simulink model "bus_io"  (Simulink 10.1)
settings: Solver=FixedStepDiscrete  StartTime=0.0  StopTime=10.0  RelTol=1e-3  EnableMultiTasking=on
settings Model: Creator=Demo  LastModifiedBy=MaximeBe
settings DataIOCC: LimitDataPoints=on  SaveFormat=Dataset
settings OptimizationCC: ZeroExternalMemoryAtStartup=off  ZeroInternalMemoryAtStartup=off  LifeSpan=auto
settings DebuggingCC: UnderspecifiedInitializationDetection=Simplified  MergeDetectMultiDrivingBlocksExec=error  AllowSymbolicDim=off  SFExecutionAtInitializationDiag=warning
settings HardwareCC: ProdBitPerPointer=64  ProdBitPerSizeT=64  ProdBitPerPtrDiffT=64  ProdLargestAtomicFloat=Float  ProdIntDivRoundTo=Zero  ProdEndianess=LittleEndian  ProdWordSize=64  ProdHWDeviceType=Intel->x86-64 (Windows64)
settings RTWCC: Description=Generate an RTMaps component embedding the model  SystemTargetFile=rtmaps.tlc  TemplateMakefile=rtmaps_default_tmf  PostCodeGenCommand=rtmaps_post_code_generation(buildInfo)  RetainRTWFile=on  TargetLang=C++
settings STFCustomTargetCC: ModelReferenceCompliant=off  ConcurrentExecutionCompliant=on  CombineOutputUpdateFcns=on  MultiInstanceERTCode=on  CodeInterfacePackaging=C++ class  CPPClassGenCompliant=on  GRTInterface=off  SystemTargetFile=rtmaps.tlc
settings GRTTargetCC: ModelReferenceCompliant=off  ParMdlRefBuildCompliant=off  CompOptLevelCompliant=off  CombineOutputUpdateFcns=on  MatFileLogging=off  MultiInstanceERTCode=on  CodeInterfacePackaging=C++ class  GRTInterface=off  UseToolchainInfoCompliant=off
settings CPPComponent: GenerateDestructor=on  ExternalIOMemberVisibility=private  GenerateExternalIOAccessMethods=Inlined structure-based method  ParameterMemberVisibility=public  InternalMemberVisibility=private  GenerateParameterAccessMethods=None  GenerateInternalMemberAccessMethods=None  UseOperatorNewForModelRefRegistration=off  IncludeModelTypesInModelClass=on

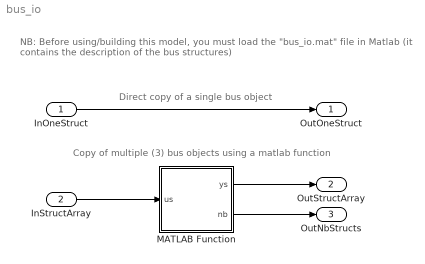
== system bus_io ==
  note: NB: Before using/building this model, you must load the "bus_io.mat"
      | file in Matlab (it contains the description of the bus structures)
  note: Copy of multiple (3) bus objects using a matlab function
  note: Direct copy of a single bus object
  InOneStruct : Inport  OutDataTypeStr=Bus: MyStruct  PortDimensions=1  BusOutputAsStruct=on
  InStructArray : Inport  Port=2  OutDataTypeStr=Bus: MyStruct  PortDimensions=3  BusOutputAsStruct=on
  MATLAB Function : MATLAB Function  TreatAsAtomicUnit=on
  OutOneStruct : Outport
  OutStructArray : Outport  Port=2
  OutNbStructs : Outport  Port=3
  wires:
  InOneStruct/1 -> OutOneStruct/1
  InStructArray/1 -> MATLAB Function/1(us)
  MATLAB Function/1(ys) -> OutStructArray/1
  MATLAB Function/2(nb) -> OutNbStructs/1

== matlab function MATLAB Function ==
  data: us input double; ys output Bus: MyStruct =0; nb output double
function [ys, nb] = fcn(us)
%#codegen

% Example of manipulating an array of one or multiple structs.
% Make sure to configure ys type in the "Edit Data" editor
% (look up the "Edit Data" button in the Toolstrip above ^)

nb = uint32(length(us));

ys = repmat(us(1), 1, nb);  % init: appears to be required

for i=1:nb

    ys(i).x = us(i).x;
    ys(i).y = us(i).y;

    l = length(us(i).arr);
    ys(i).arr = zeros(l, 1, 'int32');  % init: appears to be required
    ys(i).arr(1:l) = us(i).arr(1:l);

    ys(i).obj.a = us(i).obj.a;
    ys(i).obj.b = us(i).obj.b;

end
